simulink model "consigne_couple"  (R2024b)
settings: Solver=VariableStepAuto  StartTime=0.0  StopTime=10.0  RelTol=1e-3
undefined symbols (not defined in the file): G, Tr, w_wheels
settings Model: Creator=marti  LastModifiedBy=marti

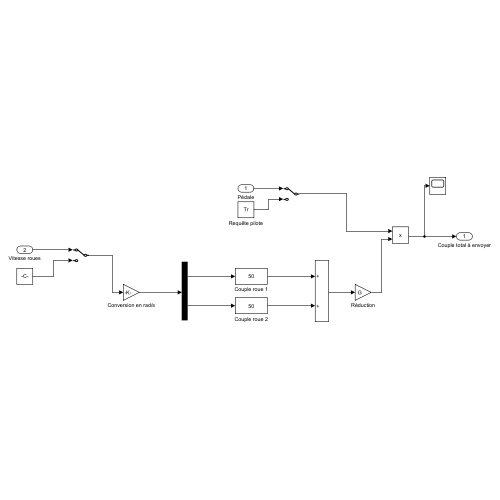
[thumbnail: Simulink's stored preview of the top-level diagram]
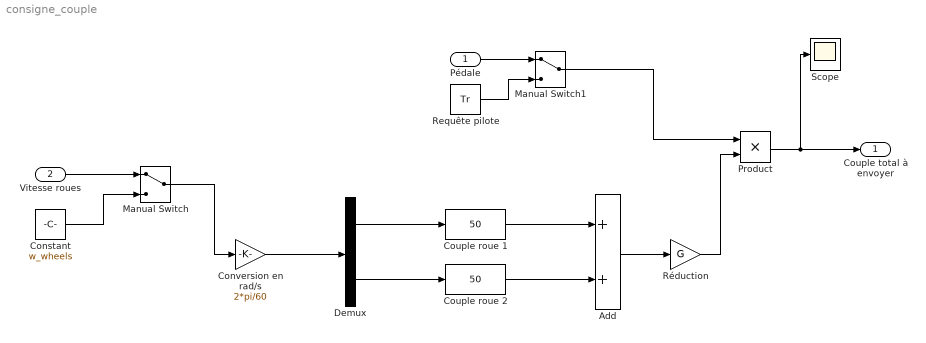
== system consigne_couple ==
  Pédale : Inport
  Vitesse roues : Inport  Port=2  PortDimensions=2
  Add : Sum
  Constant : Constant  Value=w_wheels
  Conversion en rad/s : Gain  Gain=2*pi/60
  Couple roue 1 : Fcn  Expr=50
  Couple roue 2 : Fcn  Expr=50
  Demux : Demux  Outputs=2
  Manual Switch : ManualSwitch
  Manual Switch1 : ManualSwitch
  Product : Product
  Requête pilote : Constant  Value=Tr
  Réduction : Gain  Gain=G
  Scope : Scope
  Couple total à envoyer : Outport
  wires:
  Add/1 -> Réduction/1
  Réduction/1 -> Product/2
  Pédale/1 -> Manual Switch1/1
  Requête pilote/1 -> Manual Switch1/2
  Manual Switch1/1 -> Product/1
  Product/1 -> Scope/1, Couple total à envoyer/1
  Conversion en rad/s/1 -> Demux/1
  Constant/1 -> Manual Switch/2
  Manual Switch/1 -> Conversion en rad/s/1
  Vitesse roues/1 -> Manual Switch/1
  Demux/1 -> Couple roue 1/1
  Demux/2 -> Couple roue 2/1
  Couple roue 1/1 -> Add/1
  Couple roue 2/1 -> Add/2
